simulink model "threephase_separateHbridge"  (R2018a)
settings: Solver=VariableStepAuto  StartTime=0.0  StopTime=0.02  MaxStep=1e-7  RelTol=1e-8
values from neighbouring files (symbols this model uses):
  M = [M11 M12; M12' M22]    [Mutual_inductance_Models_Run.m]
  R = [R11 R12;R12' R22]    [Mutual_inductance_Models_Run.m]
libraries: powerlib x72
settings Model: Creator=user  LastModifiedBy=user

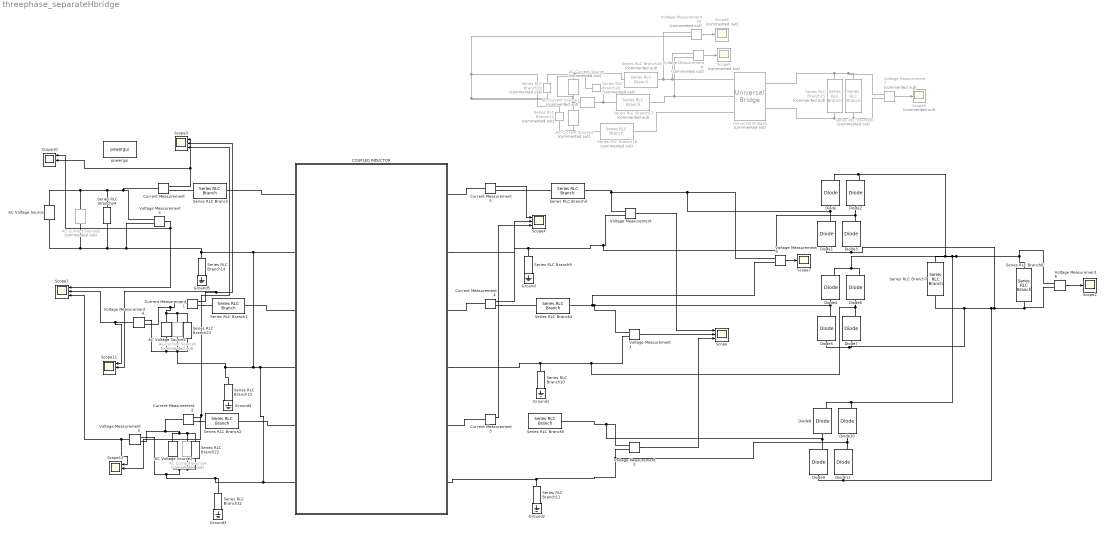
== system threephase_separateHbridge ==
  AC Current Source : powerlib/Electrical Sources/AC Current Source  Commented=on  Amplitude=10  Phase=0  Frequency=200000  SampleTime=0  Measurements=None
      settings: SourceProductName=Simscape Power Systems  SourceProductBaseCode=PS
  AC Current Source1 : powerlib/Electrical Sources/AC Current Source  Commented=on  Amplitude=10  Phase=240  Frequency=200000  SampleTime=0  Measurements=None
      settings: SourceProductName=Simscape Power Systems  SourceProductBaseCode=PS
  AC Current Source2 : powerlib/Electrical Sources/AC Current Source  Commented=on  Amplitude=10  Phase=120  Frequency=200000  SampleTime=0  Measurements=None
      settings: SourceProductName=Simscape Power Systems  SourceProductBaseCode=PS
  AC Current Source4 : powerlib/Electrical Sources/AC Current Source  Commented=on  Amplitude=10  Phase=240  Frequency=200000  SampleTime=0  Measurements=None
      settings: SourceProductName=Simscape Power Systems  SourceProductBaseCode=PS
  AC Current Source5 : powerlib/Electrical Sources/AC Current Source  Commented=on  Amplitude=10  Phase=0  Frequency=200000  SampleTime=0  Measurements=None
      settings: SourceProductName=Simscape Power Systems  SourceProductBaseCode=PS
  AC Current Source6 : powerlib/Electrical Sources/AC Current Source  Commented=on  Amplitude=10  Phase=0  Frequency=200000  SampleTime=0  Measurements=None
      settings: SourceProductName=Simscape Power Systems  SourceProductBaseCode=PS
  AC Voltage Source : powerlib/Electrical Sources/AC Voltage Source  Amplitude=100  Phase=0  Frequency=200000  SampleTime=0  Measurements=None  BusType=swing  Pref=10e3  Qref=0  Qmin=-inf  Qmax=+inf
  AC Voltage Source1 : powerlib/Electrical Sources/AC Voltage Source  Amplitude=100  Phase=120  Frequency=200000  SampleTime=0  Measurements=None  BusType=swing  Pref=10e3  Qref=0  Qmin=-inf  Qmax=+inf
  AC Voltage Source2 : powerlib/Electrical Sources/AC Voltage Source  Amplitude=100  Phase=240  Frequency=200000  SampleTime=0  Measurements=None  BusType=swing  Pref=10e3  Qref=0  Qmin=-inf  Qmax=+inf
  COUPLED INDUCTOR : Subsystem
  Current Measurement{,1..5} (6 alike) : powerlib/Measurements/Current Measurement  PhasorSimulation=off  OutputType=Complex  PSBequivalent=0
  Diode{,1..11} (12 alike) : powerlib/Power Electronics/Diode  Ron=0.001  Lon=0  Vf=0.8  IC=0  UseSnubber=0  Rs=inf  Cs=250e-9  Measurements=on
  Ground{,1..5} (6 alike) : powerlib/Elements/Ground  LConnTagsString=a
  Scope{,1,3..4,10..12} (7 alike) : Scope  NumInputPorts=3
  Scope2 : Scope
  Scope5 : Scope  Commented=on
  Scope6 : Scope  Commented=on
  Scope7 : Scope
  Scope8 : Scope  Commented=on
  Series RLC Branch : powerlib/Elements/Series RLC Branch  LConnTagsString=__new0  RConnTagsString=__new0  BranchType=C  Resistance=1  Inductance=1e-3  SetiL0=off  InitialCurrent=0  Capacitance=7.7e-9  Setx0=off  InitialVoltage=0  Measurements=None
  Series RLC Branch1 : powerlib/Elements/Series RLC Branch  LConnTagsString=__new0  RConnTagsString=__new0  BranchType=C  Resistance=1  Inductance=1e-3  SetiL0=off  InitialCurrent=0  Capacitance=7.7e-9  Setx0=off  InitialVoltage=0  Measurements=None
  Series RLC Branch{9..14,22..24} (9 alike) : powerlib/Elements/Series RLC Branch  LConnTagsString=__new0  RConnTagsString=__new0  BranchType=R  Resistance=10000  Inductance=1e-3  SetiL0=off  InitialCurrent=0  Capacitance=9.95e-9  Setx0=off  InitialVoltage=0  Measurements=None
  Series RLC Branch15 : powerlib/Elements/Series RLC Branch  Commented=on  LConnTagsString=__new0  RConnTagsString=__new0  BranchType=C  Resistance=30  Inductance=1e-3  SetiL0=off  InitialCurrent=0  Capacitance=1e-6  Setx0=off  InitialVoltage=0  Measurements=None
  Series RLC Branch16 : powerlib/Elements/Series RLC Branch  Commented=on  LConnTagsString=__new0  RConnTagsString=__new0  BranchType=R  Resistance=1  Inductance=1e-3  SetiL0=off  InitialCurrent=0  Capacitance=9.95e-9  Setx0=off  InitialVoltage=0  Measurements=None
  Series RLC Branch17 : powerlib/Elements/Series RLC Branch  Commented=on  LConnTagsString=__new0  RConnTagsString=__new0  BranchType=R  Resistance=1  Inductance=1e-3  SetiL0=off  InitialCurrent=0  Capacitance=9.95e-9  Setx0=off  InitialVoltage=0  Measurements=None
  Series RLC Branch18 : powerlib/Elements/Series RLC Branch  Commented=on  LConnTagsString=__new0  RConnTagsString=__new0  BranchType=R  Resistance=1  Inductance=1e-3  SetiL0=off  InitialCurrent=0  Capacitance=9.95e-9  Setx0=off  InitialVoltage=0  Measurements=None
  Series RLC Branch19 : powerlib/Elements/Series RLC Branch  Commented=on  LConnTagsString=__new0  RConnTagsString=__new0  BranchType=R  Resistance=10000  Inductance=1e-3  SetiL0=off  InitialCurrent=0  Capacitance=9.95e-9  Setx0=off  InitialVoltage=0  Measurements=None
  Series RLC Branch2 : powerlib/Elements/Series RLC Branch  LConnTagsString=__new0  RConnTagsString=__new0  BranchType=C  Resistance=1  Inductance=1e-3  SetiL0=off  InitialCurrent=0  Capacitance=7.7e-9  Setx0=off  InitialVoltage=0  Measurements=None
  Series RLC Branch20 : powerlib/Elements/Series RLC Branch  Commented=on  LConnTagsString=__new0  RConnTagsString=__new0  BranchType=R  Resistance=10000  Inductance=1e-3  SetiL0=off  InitialCurrent=0  Capacitance=9.95e-9  Setx0=off  InitialVoltage=0  Measurements=None
  Series RLC Branch21 : powerlib/Elements/Series RLC Branch  Commented=on  LConnTagsString=__new0  RConnTagsString=__new0  BranchType=R  Resistance=10000  Inductance=1e-3  SetiL0=off  InitialCurrent=0  Capacitance=9.95e-9  Setx0=off  InitialVoltage=0  Measurements=None
  Series RLC Branch3 : powerlib/Elements/Series RLC Branch  LConnTagsString=__new0  RConnTagsString=__new0  BranchType=C  Resistance=1  Inductance=1e-3  SetiL0=off  InitialCurrent=0  Capacitance=9.95e-9  Setx0=off  InitialVoltage=0  Measurements=None
  Series RLC Branch4 : powerlib/Elements/Series RLC Branch  LConnTagsString=__new0  RConnTagsString=__new0  BranchType=C  Resistance=1  Inductance=1e-3  SetiL0=off  InitialCurrent=0  Capacitance=9.95e-9  Setx0=off  InitialVoltage=0  Measurements=None
  Series RLC Branch5 : powerlib/Elements/Series RLC Branch  LConnTagsString=__new0  RConnTagsString=__new0  BranchType=C  Resistance=1  Inductance=1e-3  SetiL0=off  InitialCurrent=0  Capacitance=9.95e-9  Setx0=off  InitialVoltage=0  Measurements=None
  Series RLC Branch6 : powerlib/Elements/Series RLC Branch  LConnTagsString=__new0  RConnTagsString=__new0  BranchType=R  Resistance=30  Inductance=1e-3  SetiL0=off  InitialCurrent=0  Capacitance=9.95e-9  Setx0=off  InitialVoltage=0  Measurements=None
  Series RLC Branch7 : powerlib/Elements/Series RLC Branch  LConnTagsString=__new0  RConnTagsString=__new0  BranchType=C  Resistance=30  Inductance=1e-3  SetiL0=off  InitialCurrent=0  Capacitance=1e-6  Setx0=off  InitialVoltage=0  Measurements=None
  Series RLC Branch8 : powerlib/Elements/Series RLC Branch  Commented=on  LConnTagsString=__new0  RConnTagsString=__new0  BranchType=R  Resistance=30  Inductance=1e-3  SetiL0=off  InitialCurrent=0  Capacitance=9.95e-9  Setx0=off  InitialVoltage=0  Measurements=None
  Universal Bridge1 : powerlib/Power Electronics/Universal Bridge  Commented=on  Arms=3  SnubberResistance=inf  SnubberCapacitance=inf  Device=Diodes  Ron=1e-3  Lon=0  ForwardVoltages="[  0  0  ]"  ForwardVoltage=0  GTOparameters=[ 10e-6 , 20e-6 ]  IGBTparameters=[ 1e-6 , 2e-6 ]  Measurements=None  Measurements_2=None  converterType=Rectifier
  Voltage Measurement{,1..6,9} (8 alike) : powerlib/Measurements/Voltage Measurement  PhasorSimulation=off  OutputType=Complex  PSBequivalent=0
  Voltage Measurement10 : powerlib/Measurements/Voltage Measurement  Commented=on  PhasorSimulation=off  OutputType=Complex  PSBequivalent=0
  Voltage Measurement7 : powerlib/Measurements/Voltage Measurement  Commented=on  PhasorSimulation=off  OutputType=Complex  PSBequivalent=0
  Voltage Measurement8 : powerlib/Measurements/Voltage Measurement  Commented=on  PhasorSimulation=off  OutputType=Complex  PSBequivalent=0
  powergui : powerlib/powergui  Priority=1  SimulationMode=Continuous  SampleTime=50e-6  frequency=60  Iterations=50  frequencyindice=200000  Pbase=100e6  ErrMax=1e-4  UnitsV=kV  UnitsW=MW  buscounter=0  FunctionMessages=off  echomessages=off  EnableUseOfTLC=off  CurrentSourceSwitches=off  DisableSnubberDevices=off  DisableRonSwitches=off  DisableVfSwitches=off  DisplayEquations=off  SolverType=Tustin/Backward Euler (TBE)  Interpol=off  ExternalGateDelay=off  methode=off  Ts=100  x0status=blocks  SPID=on  SwTol=0  HookPort=off  RestoreLinks=warning  ResistiveCurrentMeasurement=off  Frange=[0:2:500]  Ylog=off  Xlog=on  ShowGrid=off  save=off  variable=ZData  structure=0  ZoomFFT=off  StartTime=0.0  cycles=1  DisplayStyle=1  fundamental=60  FreqAxis=off  MaxFrequency=1000  frequencyindicesteady=1  RmsSteady=1  display=off
  wires:
  Voltage Measurement/1 -> Scope/1
  Voltage Measurement1/1 -> Scope/2
  Voltage Measurement2/1 -> Scope/3
  Voltage Measurement3/1 -> Scope10/1, Scope1/1
  Voltage Measurement4/1 -> Scope11/1, Scope1/2
  Voltage Measurement5/1 -> Scope12/1, Scope1/3
  Voltage Measurement6/1 -> Scope2/1
  Current Measurement/1 -> Scope10/2, Scope3/1
  Current Measurement1/1 -> Scope11/2, Scope3/2
  Current Measurement2/1 -> Scope12/2, Scope3/3
  Current Measurement5/1 -> Scope4/1
  Current Measurement4/1 -> Scope4/2
  Current Measurement3/1 -> Scope4/3
  Voltage Measurement7/1 -> Scope5/1
  Voltage Measurement8/1 -> Scope6/1
  Voltage Measurement9/1 -> Scope7/1
  Voltage Measurement10/1 -> Scope8/1
  connections:
  Voltage Measurement3/LConn1 -- Series RLC Branch24/LConn1 -- AC Current Source6/RConn1 -- AC Voltage Source/RConn1 -- Current Measurement/LConn1
  Voltage Measurement4/LConn1 -- Current Measurement1/LConn1 -- Series RLC Branch23/LConn1 -- AC Current Source5/RConn1 -- AC Voltage Source1/RConn1
  Voltage Measurement5/LConn1 -- Series RLC Branch22/LConn1 -- AC Current Source4/RConn1 -- AC Voltage Source2/RConn1 -- Current Measurement2/LConn1
  Series RLC Branch14/LConn1 -- AC Current Source4/LConn1 -- Series RLC Branch22/RConn1 -- AC Voltage Source2/LConn1 -- Voltage Measurement5/LConn2 -- Series RLC Branch12/LConn1 -- COUPLED INDUCTOR/RConn6 -- COUPLED INDUCTOR/RConn4 -- Voltage Measurement4/LConn2 -- AC Current Source5/LConn1 -- AC Voltage Source1/LConn1 -- Series RLC Branch23/RConn1 -- Series RLC Branch13/LConn1 -- COUPLED INDUCTOR/RConn2 -- AC Current Source6/LConn1 -- AC Voltage Source/LConn1 -- Series RLC Branch24/RConn1 -- Voltage Measurement3/LConn2
  Diode2/LConn1 -- COUPLED INDUCTOR/LConn2 -- Series RLC Branch9/LConn1 -- Voltage Measurement/LConn2 -- Diode3/RConn1
  COUPLED INDUCTOR/RConn1 -- Series RLC Branch/RConn1
  COUPLED INDUCTOR/RConn3 -- Series RLC Branch1/RConn1
  COUPLED INDUCTOR/RConn5 -- Series RLC Branch2/RConn1
  Current Measurement/RConn1 -- Series RLC Branch/LConn1
  Current Measurement1/RConn1 -- Series RLC Branch1/LConn1
  Current Measurement2/RConn1 -- Series RLC Branch2/LConn1
  Current Measurement5/LConn1 -- COUPLED INDUCTOR/LConn1
  Current Measurement5/RConn1 -- Series RLC Branch3/LConn1
  Current Measurement4/RConn1 -- Series RLC Branch4/LConn1
  Current Measurement4/LConn1 -- COUPLED INDUCTOR/LConn3
  Current Measurement3/LConn1 -- COUPLED INDUCTOR/LConn5
  AC Current Source/LConn1 -- Series RLC Branch21/RConn1 -- Voltage Measurement10/LConn2 -- Series RLC Branch19/LConn1 -- Series RLC Branch20/LConn1 -- AC Current Source2/LConn1 -- AC Current Source1/LConn1
  AC Current Source2/RConn1 -- Series RLC Branch21/LConn1 -- Series RLC Branch18/RConn1
  AC Current Source1/RConn1 -- Series RLC Branch20/RConn1 -- Series RLC Branch17/RConn1
  Series RLC Branch16/LConn1 -- Voltage Measurement10/LConn1 -- Voltage Measurement8/LConn1 -- Universal Bridge1/LConn1
  Voltage Measurement7/LConn1 -- Series RLC Branch8/LConn1 -- Universal Bridge1/RConn1 -- Series RLC Branch15/LConn1
  Voltage Measurement7/LConn2 -- Series RLC Branch8/RConn1 -- Universal Bridge1/RConn2 -- Series RLC Branch15/RConn1
  AC Current Source/RConn1 -- Series RLC Branch19/RConn1 -- Series RLC Branch16/RConn1
  Series RLC Branch17/LConn1 -- Voltage Measurement8/LConn2 -- Universal Bridge1/LConn2
  Series RLC Branch18/LConn1 -- Universal Bridge1/LConn3
  Diode4/LConn1 -- Voltage Measurement9/LConn2 -- Series RLC Branch4/RConn1 -- Voltage Measurement1/LConn1 -- Diode5/RConn1
  Diode/LConn1 -- Series RLC Branch3/RConn1 -- Voltage Measurement/LConn1 -- Voltage Measurement9/LConn1 -- Diode1/RConn1
  Diode6/LConn1 -- COUPLED INDUCTOR/LConn4 -- Series RLC Branch10/LConn1 -- Voltage Measurement1/LConn2 -- Diode7/RConn1
  Diode10/LConn1 -- COUPLED INDUCTOR/LConn6 -- Series RLC Branch11/LConn1 -- Voltage Measurement2/LConn2 -- Diode11/RConn1
  Voltage Measurement2/LConn1 -- Diode8/LConn1 -- Diode9/RConn1 -- Series RLC Branch5/RConn1
  Diode7/LConn1 -- Diode9/LConn1 -- Diode11/LConn1 -- Diode1/LConn1 -- Diode3/LConn1 -- Voltage Measurement6/LConn2 -- Series RLC Branch6/RConn1 -- Series RLC Branch7/RConn1 -- Diode5/LConn1
  Diode6/RConn1 -- Diode8/RConn1 -- Diode10/RConn1 -- Diode/RConn1 -- Diode2/RConn1 -- Series RLC Branch7/LConn1 -- Series RLC Branch6/LConn1 -- Voltage Measurement6/LConn1 -- Diode4/RConn1

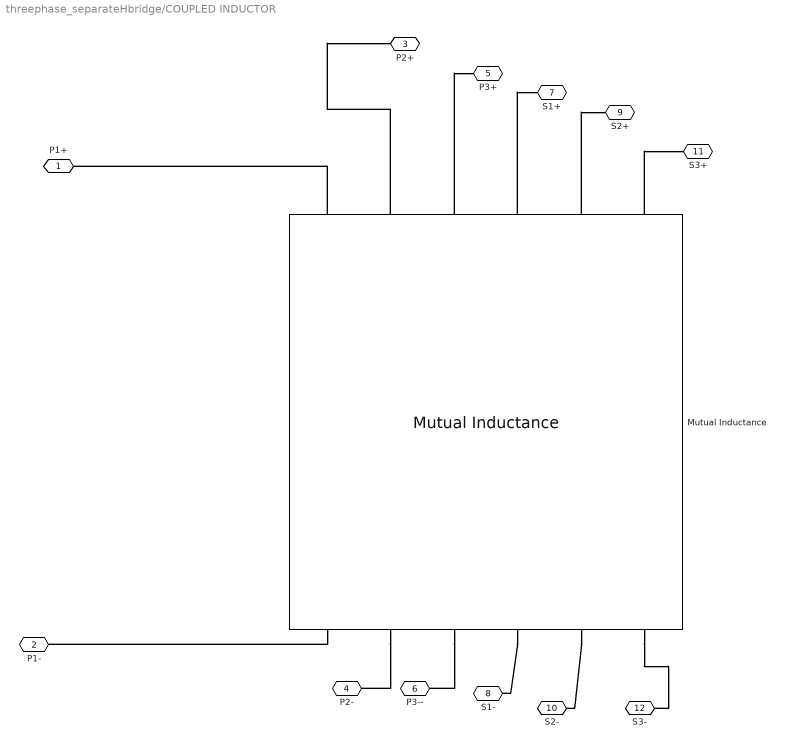
== system threephase_separateHbridge/COUPLED INDUCTOR ==
  Mutual Inductance : powerlib/Elements/Mutual Inductance  LConnTagsString=a|b|c|L4|L5|L6  RConnTagsString=A|B|C|R4|R5|R6  TypeOfMutual=Generalized mutual inductance  NumberOfWindings=6  SelfImpedance1=[1.1 1.1e-03]  SelfImpedance2=[ 1.1 1.1e-03]  ThreeWindings=on  SelfImpedance3=[ 1.1 1.1e-03]  MutualImpedance=[1.0 1.0e-03]  InductanceMatrix=M * 1e-6  ResistanceMatrix=R*0.001  Measurements=None
      settings: AttributesFormatString=\n  SourceProductName=Simscape Power Systems  SourceProductBaseCode=PS
  P1+ : PMIOPort  Side=Right
  P1- : PMIOPort  Port=2  Side=Right
  P2+ : PMIOPort  Port=3  Side=Right
  P2- : PMIOPort  Port=4  Side=Right
  P3+ : PMIOPort  Port=5  Side=Right
  P3-- : PMIOPort  Port=6  Side=Right
  S1+ : PMIOPort  Port=7  Side=Left
  S1- : PMIOPort  Port=8  Side=Left
  S2+ : PMIOPort  Port=9  Side=Left
  S2- : PMIOPort  Port=10  Side=Left
  "S3+ " : PMIOPort  Port=11  Side=Left
  "S3- " : PMIOPort  Port=12  Side=Left
  connections:
  Mutual Inductance/LConn2 -- P2-/RConn1
  Mutual Inductance/LConn5 -- S2-/RConn1
  Mutual Inductance/RConn5 -- S2+/RConn1
  Mutual Inductance/RConn4 -- S1+/RConn1
  Mutual Inductance/LConn6 -- "S3- "/RConn1
  Mutual Inductance/RConn1 -- P1+/RConn1
  Mutual Inductance/LConn1 -- P1-/RConn1
  Mutual Inductance/RConn2 -- P2+/RConn1
  Mutual Inductance/LConn4 -- S1-/RConn1
  Mutual Inductance/LConn3 -- P3--/RConn1
  Mutual Inductance/RConn3 -- P3+/RConn1
  Mutual Inductance/RConn6 -- "S3+ "/RConn1
